simulink model "CustomBlockFullTest"  (R2015b)
settings: Solver=VariableStepAuto  StartTime=0.0  StopTime=inf  RelTol=1e-3
libraries: MonitoringSystem x18, aerolibanimutils x1, simulink x1, dspnetwork x1
settings Model: Creator=Ryuu  LastModifiedBy=Ryuu

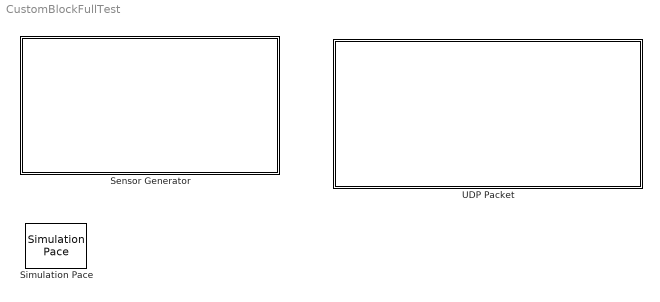
== system CustomBlockFullTest ==
  "Sensor Generator " : Subsystem
  Simulation Pace : aerolibanimutils/Simulation Pace  SimulationPace=1  SleepMode=MATLAB Thread  OutputPaceError=off  SampleTime=1/30
  UDP Packet : Subsystem

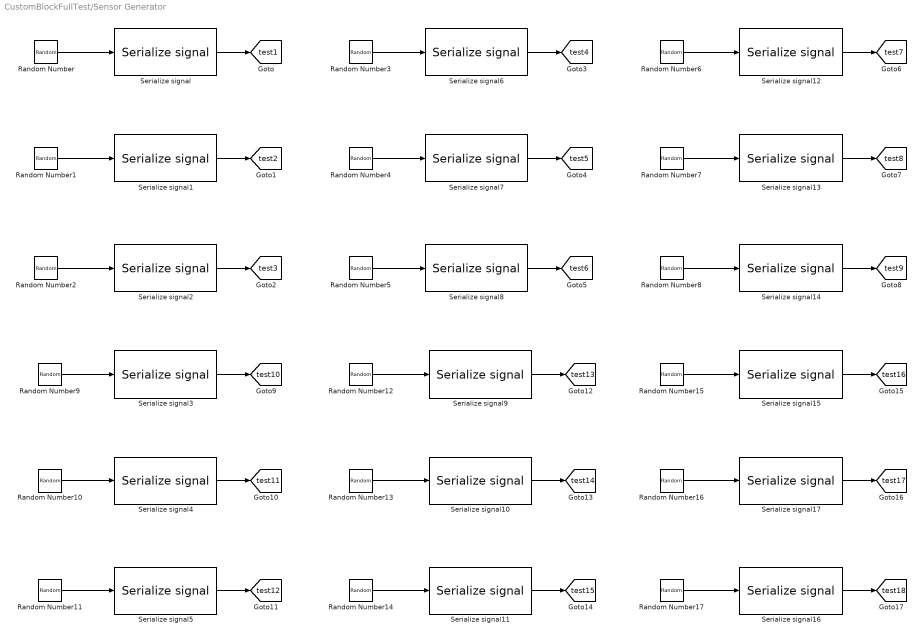
== system CustomBlockFullTest/Sensor Generator  ==
  Random Number : RandomNumber  Mean=100  Variance=50  Seed=1  SampleTime=0.02
  Random Number1 : RandomNumber  Mean=100  Variance=50  Seed=2  SampleTime=0.02
  Random Number10 : RandomNumber  Mean=100  Variance=50  Seed=11  SampleTime=0.02
  Random Number11 : RandomNumber  Mean=100  Variance=50  Seed=12  SampleTime=0.02
  Random Number12 : RandomNumber  Mean=100  Variance=50  Seed=13  SampleTime=0.02
  Random Number13 : RandomNumber  Mean=100  Variance=50  Seed=14  SampleTime=0.02
  Random Number14 : RandomNumber  Mean=100  Variance=50  Seed=15  SampleTime=0.02
  Random Number15 : RandomNumber  Mean=100  Variance=50  Seed=16  SampleTime=0.02
  Random Number16 : RandomNumber  Mean=100  Variance=50  Seed=17  SampleTime=0.02
  Random Number17 : RandomNumber  Mean=100  Variance=50  Seed=18  SampleTime=0.02
  Random Number2 : RandomNumber  Mean=100  Variance=50  Seed=3  SampleTime=0.02
  Random Number3 : RandomNumber  Mean=100  Variance=50  Seed=4  SampleTime=0.02
  Random Number4 : RandomNumber  Mean=100  Variance=50  Seed=5  SampleTime=0.02
  Random Number5 : RandomNumber  Mean=100  Variance=50  Seed=6  SampleTime=0.02
  Random Number6 : RandomNumber  Mean=100  Variance=50  Seed=7  SampleTime=0.02
  Random Number7 : RandomNumber  Mean=100  Variance=50  Seed=8  SampleTime=0.02
  Random Number8 : RandomNumber  Mean=100  Variance=50  Seed=9  SampleTime=0.02
  Random Number9 : RandomNumber  Mean=100  Variance=50  Seed=10  SampleTime=0.02
  Serialize signal : MonitoringSystem/Serialize signal  label='Test 1'  signal_type=Type a  min=0  max=100
  Serialize signal1 : MonitoringSystem/Serialize signal  label='Test 2'  signal_type=Type d  min=5  max=28
  Serialize signal10 : MonitoringSystem/Serialize signal  label='Test 14'  signal_type=Type b  min=34  max=3213
  Serialize signal11 : MonitoringSystem/Serialize signal  label='Test 15'  signal_type=Type m  min=0  max=453
  Serialize signal12 : MonitoringSystem/Serialize signal  label='Test 7'  signal_type=Type l  min=0  max=100
  Serialize signal13 : MonitoringSystem/Serialize signal  label='Test 8'  signal_type=Type k  min=14  max=74
  Serialize signal14 : MonitoringSystem/Serialize signal  label='Test 9'  signal_type=Type f  min=456  max=8907
  Serialize signal15 : MonitoringSystem/Serialize signal  label='Test 16'  signal_type=Type j  min=0  max=100
  Serialize signal16 : MonitoringSystem/Serialize signal  label='Test 18'  signal_type=Type k  min=0  max=98
  Serialize signal17 : MonitoringSystem/Serialize signal  label='Test 17'  signal_type=Type k  min=45  max=2146
  Serialize signal2 : MonitoringSystem/Serialize signal  label='Test 3'  signal_type=Type i  min=8  max=400
  Serialize signal3 : MonitoringSystem/Serialize signal  label='Test 10'  signal_type=Type l  min=0  max=24
  Serialize signal4 : MonitoringSystem/Serialize signal  label='Test 11'  signal_type=Type m  min=2  max=8765
  Serialize signal5 : MonitoringSystem/Serialize signal  label='Test 12'  signal_type=Type j  min=0  max=867
  Serialize signal6 : MonitoringSystem/Serialize signal  label='Test 4'  signal_type=Type h  min=1  max=2
  Serialize signal7 : MonitoringSystem/Serialize signal  label='Test 5'  signal_type=Type l  min=0  max=76
  Serialize signal8 : MonitoringSystem/Serialize signal  label='Test 6'  signal_type=Type g  min=1  max=2
  Serialize signal9 : MonitoringSystem/Serialize signal  label='Test 13'  signal_type=Type b  min=0  max=567
  tag scope: test10=global, test11=global, test12=global, test13=global, test14=global, test15=global, test16=global, test17=global, test18=global, test1=global, test2=global, test3=global, test4=global, test5=global, test6=global, test7=global, test8=global, test9=global
  wires:
  Random Number/1 -> Serialize signal/1
  Serialize signal/1 -> [test1]
  Random Number1/1 -> Serialize signal1/1
  Serialize signal1/1 -> [test2]
  Random Number2/1 -> Serialize signal2/1
  Serialize signal2/1 -> [test3]
  Random Number3/1 -> Serialize signal6/1
  Serialize signal6/1 -> [test4]
  Random Number4/1 -> Serialize signal7/1
  Serialize signal7/1 -> [test5]
  Random Number5/1 -> Serialize signal8/1
  Serialize signal8/1 -> [test6]
  Random Number6/1 -> Serialize signal12/1
  Serialize signal12/1 -> [test7]
  Random Number7/1 -> Serialize signal13/1
  Serialize signal13/1 -> [test8]
  Random Number8/1 -> Serialize signal14/1
  Serialize signal14/1 -> [test9]
  Random Number9/1 -> Serialize signal3/1
  Serialize signal3/1 -> [test10]
  Random Number10/1 -> Serialize signal4/1
  Serialize signal4/1 -> [test11]
  Random Number11/1 -> Serialize signal5/1
  Serialize signal5/1 -> [test12]
  Random Number12/1 -> Serialize signal9/1
  Serialize signal9/1 -> [test13]
  Random Number13/1 -> Serialize signal10/1
  Serialize signal10/1 -> [test14]
  Random Number14/1 -> Serialize signal11/1
  Serialize signal11/1 -> [test15]
  Random Number15/1 -> Serialize signal15/1
  Serialize signal15/1 -> [test16]
  Random Number16/1 -> Serialize signal17/1
  Random Number17/1 -> Serialize signal16/1
  Serialize signal16/1 -> [test18]
  Serialize signal17/1 -> [test17]

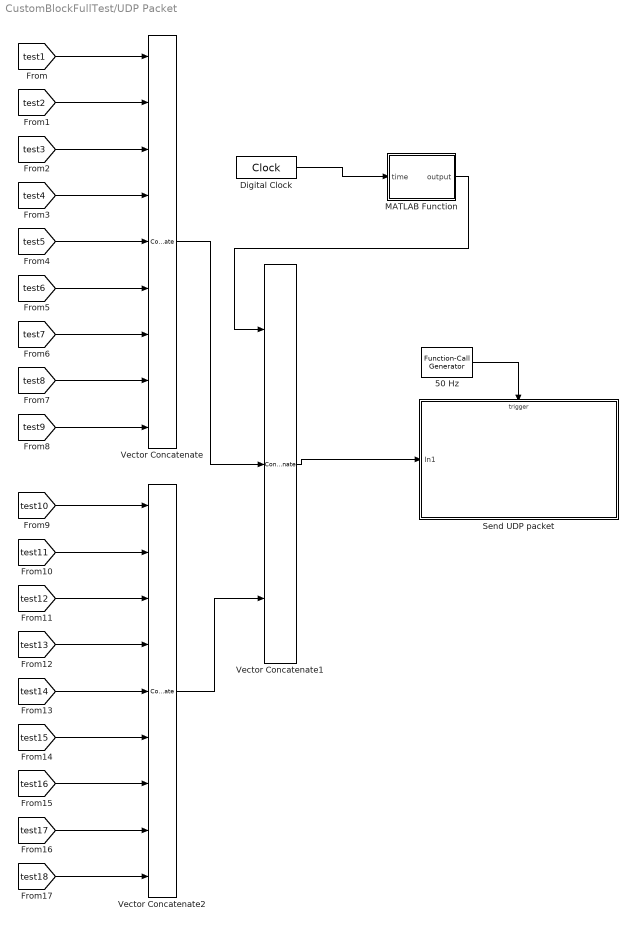
== system CustomBlockFullTest/UDP Packet ==
  50 Hz : simulink/Ports & Subsystems/Function-Call Generator  sample_time=0.02  numberOfIterations=1
  Digital Clock : DigitalClock  SampleTime=0.001
  MATLAB Function : MATLAB Function  TreatAsAtomicUnit=on
  Send UDP packet : Subsystem
  Vector Concatenate : Concatenate  NumInputs=9
  Vector Concatenate1 : Concatenate  NumInputs=3
  Vector Concatenate2 : Concatenate  NumInputs=9
  wires:
  [test1] -> Vector Concatenate/1
  50 Hz/1 -> Send UDP packet/Trigger
  [test2] -> Vector Concatenate/2
  [test3] -> Vector Concatenate/3
  [test4] -> Vector Concatenate/4
  [test5] -> Vector Concatenate/5
  [test6] -> Vector Concatenate/6
  [test7] -> Vector Concatenate/7
  [test8] -> Vector Concatenate/8
  [test9] -> Vector Concatenate/9
  [test10] -> Vector Concatenate2/1
  [test11] -> Vector Concatenate2/2
  [test12] -> Vector Concatenate2/3
  [test13] -> Vector Concatenate2/4
  [test14] -> Vector Concatenate2/5
  [test15] -> Vector Concatenate2/6
  [test16] -> Vector Concatenate2/7
  [test17] -> Vector Concatenate2/8
  [test18] -> Vector Concatenate2/9
  Vector Concatenate1/1 -> Send UDP packet/1(In1)
  Digital Clock/1 -> MATLAB Function/1(time)
  MATLAB Function/1(output) -> Vector Concatenate1/1
  Vector Concatenate/1 -> Vector Concatenate1/2
  Vector Concatenate2/1 -> Vector Concatenate1/3

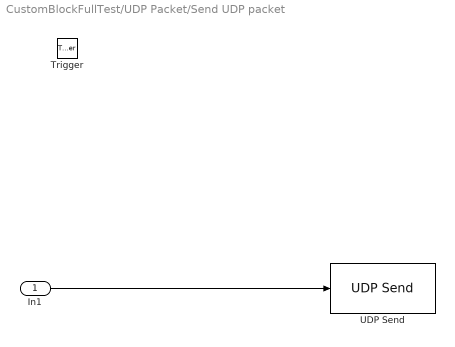
== system CustomBlockFullTest/UDP Packet/Send UDP packet ==
  In1 : Inport
  Trigger : TriggerPort  TriggerType=function-call  PortDimensions=1
  UDP Send : dspnetwork/UDP Send  remoteURL='127.0.0.1'  remotePort=25000  localURL='0.0.0.0'  localPortSource=Automatically determine  localPort=-1  sampletime=-1  separateLengthPort=0
  wires:
  In1/1 -> UDP Send/1

== matlab function CustomBlockFullTest/UDP Packet/MATLAB Function ==
  data: time input; output output
function output = time_serialize(time)

time_ser = serialize(time);
output = time_ser;
end


function m = serialize(v)
    % dispatch according to type
    if isnumeric(v) 
        m = serialize_numeric(v);
    elseif ischar(v)
        m = serialize_string(v);
    elseif islogical(v)
        m = serialize_logical(v);
	else
		error('Unsupported data type');
    end
end

% single scalar
function m = serialize_scalar(v)
    % Data type & data
    m = [class2tag(class(v)); typecast(v,'uint8').'];
end

% char arrays
function m = serialize_string(v)
    if size(v,1) == 1
        % horizontal string: Type, Length, and Data
        m = [uint8(0); typecast(uint32(length(v)),'uint8').'; uint8(v(:))];
    elseif sum(size(v)) == 0
        % '': special encoding
        m = uint8(200);
    else
        % general char array: Tag & Number of dimensions, Dimensions, Data
        m = [uint8(132); ndims(v); typecast(uint32(size(v)),'uint8').'; uint8(v(:))];
    end
end

% logical arrays
function m = serialize_logical(v)
    % Tag & Number of dimensions, Dimensions, Data
    m = [uint8(133); ndims(v); typecast(uint32(size(v)),'uint8').'; uint8(v(:))];
end

% non-complex and non-sparse numerical matrix
function m = serialize_numeric_simple(v)
    % Tag & Number of dimensions, Dimensions, Data
    m = [16+class2tag(class(v)); ndims(v); typecast(uint32(size(v)),'uint8').'; typecast(v(:).','uint8').'];
end

% Numeric Matrix: can be real/complex, sparse/full, scalar
function m = serialize_numeric(v)
    if issparse(v)
        % Data Type & Dimensions
        m = [uint8(130); typecast(uint64(size(v,1)), 'uint8').'; typecast(uint64(size(v,2)), 'uint8').']; % vectorize
        % Index vectors
        [i,j,s] = find(v);        
        % Real/Complex
        if isreal(v)
            m = [m; serialize_numeric_simple(i); serialize_numeric_simple(j); 1; serialize_numeric_simple(s)];
        else
            m = [m; serialize_numeric_simple(i); serialize_numeric_simple(j); 0; serialize_numeric_simple(real(s)); serialize_numeric_simple(imag(s))];
        end
    elseif ~isreal(v)
        % Data type & contents
        m = [uint8(131); serialize_numeric_simple(real(v)); serialize_numeric_simple(imag(v))];
    elseif isscalar(v)
        % Scalar
        m = serialize_scalar(v);
    else
        % Simple matrix
        m = serialize_numeric_simple(v);
    end
end

% *container* class to byte
function b = class2tag(cls)
	switch cls
		case 'string'
            b = uint8(0);
		case 'double'
			b = uint8(1);
		case 'single'
			b = uint8(2);
		case 'int8'
			b = uint8(3);
		case 'uint8'
			b = uint8(4);
		case 'int16'
			b = uint8(5);
		case 'uint16'
			b = uint8(6);
		case 'int32'
			b = uint8(7);
		case 'uint32'
			b = uint8(8);
		case 'int64'
			b = uint8(9);
		case 'uint64'
			b = uint8(10);
		otherwise
			error('Unknown class');
    end
end
